simulink model "untitled1"  (R2023a)
settings: Solver=VariableStepAuto  StartTime=0.0  StopTime=100  RelTol=1e-3
settings Model: Creator=thiag  LastModifiedBy=thiag

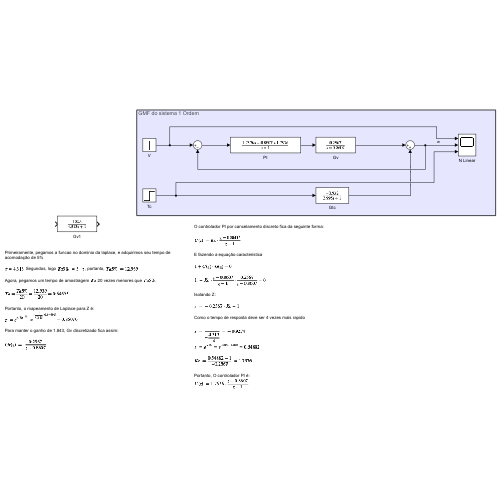
[thumbnail: Simulink's stored preview of the top-level diagram]
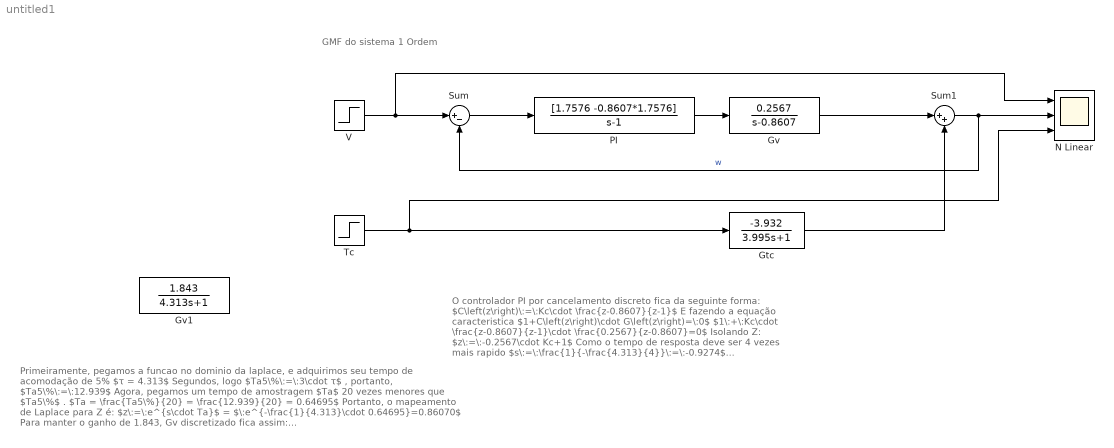
== system untitled1 ==
  note: O controlador PI por cancelamento discreto fica da seguinte forma:
      |
      | $C\left(z\right)\:=\:Kc\cdot \frac{z-0.8607}{z-1}$
      |
      | E fazendo a equação caracteristica
      |
      | $1+C\left(z\right)\cdot G\left(z\right)=\:0$
      |
      | $1\:+\:Kc\cdot \frac{z-0.8607}{z-1}\cdot \frac{0.2567}{z-0.8607}=0$
      |
      | Isolando Z:
      |
      | $z\:=\:-0.2567\cdot Kc+1$
      |
      | Como o tempo de resposta deve ser 4 vezes mais rapido
      |
      | $s\:=\:\frac{1}{-\frac{4.313}{4}}\:=\:-0.9274$
      | $z\:=\:e^{^{-s\cdot Ta}}\:=e^{^{-0.9274\cdot \:\:0.64695}}=\:0.54882$
      |
      | $Kc\:=\:\frac{0.54882-1}{-0.2567}\:=\:1.7576$
      |
      | Portanto, O controlador PI é:
      | $C\left(z\right)\:=\:1.7576\cdot \frac{z-0.8607}{z-1}$
  note: Primeiramente, pegamos a funcao no dominio da laplace, e adquirimos seu tempo de acomodação de 5%
      |
      | $τ = 4.313$ Segundos, logo $Ta5\%\:=\:3\cdot τ$ , portanto, $Ta5\%\:=\:12.939$
      |
      | Agora, pegamos um tempo de amostragem $Ta$ 20 vezes menores que $Ta5\%$ .
      |
      | $Ta = \frac{Ta5\%}{20} = \frac{12.939}{20} = 0.64695$
      |
      | Portanto, o mapeamento de Laplace para Z é:
      | $z\:=\:e^{s\cdot Ta}$ = $\:e^{-\frac{1}{4.313}\cdot 0.64695}=0.86070$
      |
      | Para manter o ganho de 1.843, Gv discretizado fica assim:
      |
      | $Gv\left(z\right)\:=\:\:\frac{0.2567}{z-0.8607}$
  note: GMF do sistema 1 Ordem
  Gtc : TransferFcn  Numerator=[-3.932]  Denominator=[3.995 1]
  Gv : TransferFcn  Numerator=[0.2567]  Denominator=[1 -0.8607]
  Gv1 : TransferFcn  Numerator=[1.843]  Denominator=[4.313 1]
  N Linear : Scope  NumInputPorts=3
  PI : TransferFcn  Numerator=[1.7576 -0.8607*1.7576]  Denominator=[1 -1]
  Sum : Sum  Inputs=|+-
  Sum1 : Sum  Inputs=|++
  Tc : Step  Time=30  After=2  SampleTime=0
  V : Step  Time=10  After=3  SampleTime=0
  wires:
  V/1 -> N Linear/1, Sum/1
  Tc/1 -> N Linear/3, Gtc/1
  Gtc/1 -> Sum1/2
  Sum1/1 -> Sum/2, N Linear/2  "w"
  Gv/1 -> Sum1/1
  PI/1 -> Gv/1
  Sum/1 -> PI/1
